simulink model "VDSE_2018b"  (R2018b)
settings: Solver=ode5  StartTime=0.0  StopTime=T_simulation  FixedStep=simulation_step_time  RelTol=1e-3
values from neighbouring files (symbols this model uses):
  A = 2    [vehicle_parameters_script.m]
  bump_height = 0    [vehicle_parameters_script.m]
  bump_length = 1    [vehicle_parameters_script.m]
  bump_time = 1    [vehicle_parameters_script.m]
  Bxf = 17.156    [BCD_Parameters.m]
  Bxr = 17.156    [BCD_Parameters.m]
  Byf = 12.71    [BCD_Parameters.m]
  Byr = 12.71    [BCD_Parameters.m]
  cd = 0.35    [vehicle_parameters_script.m]
  central_diff = 1    [vehicle_parameters_script.m]
  cF = 5000    [vehicle_parameters_script.m]
  clF = -0.15    [vehicle_parameters_script.m]
  clR = -0.20    (= -0.2)    [vehicle_parameters_script.m]
  cp_FA = 30    [vehicle_parameters_script.m]
  cp_RA = 13    [vehicle_parameters_script.m]
  cR = 5000    [vehicle_parameters_script.m]
  ctF = tireF.VERTICAL_DAMPING    [vehicle_parameters_script.m]
  ctR = tireR.VERTICAL_DAMPING    [vehicle_parameters_script.m]
  Cxf = 1.406    [BCD_Parameters.m]
  Cxr = 1.406    [BCD_Parameters.m]
  Cyf = 1.63    [BCD_Parameters.m]
  Cyr = 1.63    [BCD_Parameters.m]
  Dxf = 1.2    [BCD_Parameters.m]
  Dxr = 1.2    [BCD_Parameters.m]
  Dyf = 1.1    [BCD_Parameters.m]
  Dyr = 1.8    [BCD_Parameters.m]
  enableDriverControl = 0    [vehicle_parameters_script.m]
  enableLongDynamics = 1    [vehicle_parameters_script.m]
  enablePowertrain = 1    [vehicle_parameters_script.m]
  front_dr = 3.8    [vehicle_parameters_script.m]
  g = 9.806    [vehicle_parameters_script.m]
  Gear_numbers = [1 2 3 4 5 6]    [vehicle_parameters_script.m]
  GR = [2.9 1.8 1.3 1 0.85 0.75]    [vehicle_parameters_script.m]
  hcog = 0.5    [vehicle_parameters_script.m]
  hpc = 0.0    (= 0)    [vehicle_parameters_script.m]
  hrcF = 0.3    [vehicle_parameters_script.m]
  hrcg = (hrcF*lR+hrcR*lF)/(lF+lR)    (= 0.25108)    [vehicle_parameters_script.m]
  hrcR = 0.2    [vehicle_parameters_script.m]
  huFcog = 0.32    [vehicle_parameters_script.m]
  huRcog = 0.32    [vehicle_parameters_script.m]
  initial_gear = 1    [vehicle_parameters_script.m]
  JwF = 2.45    [vehicle_parameters_script.m]
  JwR = 2.45    [vehicle_parameters_script.m]
  Jx = 430    [vehicle_parameters_script.m]
  Jy = 1309    [vehicle_parameters_script.m]
  Jz = 1461    [vehicle_parameters_script.m]
  kF = 40000    [vehicle_parameters_script.m]
  kR = 35000    [vehicle_parameters_script.m]
  kRF = 0    [vehicle_parameters_script.m]
  kRR = 0    [vehicle_parameters_script.m]
  ktF = tireF.VERTICAL_STIFFNESS    [vehicle_parameters_script.m]
  ktR = tireR.VERTICAL_STIFFNESS    [vehicle_parameters_script.m]
  lF = 1.223    [vehicle_parameters_script.m]
  lR = l-lF    (= 1.277)    [vehicle_parameters_script.m]
  m = 1310    [vehicle_parameters_script.m]
  max_pressure = 1000    [vehicle_parameters_script.m]
  maxrpm = 4000    [vehicle_parameters_script.m]
  mF = 45    [vehicle_parameters_script.m]
  minrpm = 1500    [vehicle_parameters_script.m]
  mR = 50    [vehicle_parameters_script.m]
  output_samping_time = 0.001    [vehicle_parameters_script.m]
  phi0 = 0    [vehicle_parameters_script.m]
  phi_dot0 = 0    [vehicle_parameters_script.m]
  psi0 = 0    [vehicle_parameters_script.m]
  psi_dot0 = 0    [vehicle_parameters_script.m]
  rear_dr = 3.8    [vehicle_parameters_script.m]
  requested_speed = 100/3.6    (= 27.7777777778)    [vehicle_parameters_script.m]
  rF = tireF.UNLOADED_RADIUS    [vehicle_parameters_script.m]
  rho = 1.2    [vehicle_parameters_script.m]
  RPMME = Engine(:,1)    [vehicle_parameters_script.m]
  rR = tireR.UNLOADED_RADIUS    [vehicle_parameters_script.m]
  steer_ratio = 13.25    [vehicle_parameters_script.m]
  TFL = 0    [vehicle_parameters_script.m]
  TFR = 0    [vehicle_parameters_script.m]
  theta0 = 0    [vehicle_parameters_script.m]
  theta_dot0 = 0    [vehicle_parameters_script.m]
  TorqueME = []    [vehicle_parameters_script.m]
  TRL = 0    [vehicle_parameters_script.m]
  TRR = 0    [vehicle_parameters_script.m]
  Vx0 = 100/3.6    (= 27.7777777778)    [vehicle_parameters_script.m]
  Vy0 = 0    [vehicle_parameters_script.m]
  Vz0 = 0    [vehicle_parameters_script.m]
  wF = 1.578    [vehicle_parameters_script.m]
  wR = 1.544    [vehicle_parameters_script.m]
  x0 = 0    [vehicle_parameters_script.m]
  xcog_overall = (2*mR*xR+2*xF*mF+m*xs)/(m+2*mF+2*mR)    (= 1.23475333333)    [vehicle_parameters_script.m]
  y0 = 0    [vehicle_parameters_script.m]
  z0 = 0    [vehicle_parameters_script.m]
  zFL0 = 0    [vehicle_parameters_script.m]
  zFL_dot0 = 0    [vehicle_parameters_script.m]
  zFR0 = 0    [vehicle_parameters_script.m]
  zFR_dot0 = 0    [vehicle_parameters_script.m]
  zRL0 = 0    [vehicle_parameters_script.m]
  zRL_dot0 = 0    [vehicle_parameters_script.m]
  zRR0 = 0    [vehicle_parameters_script.m]
  zRR_dot0 = 0    [vehicle_parameters_script.m]
undefined symbols (not defined in the file or in its folder): exf, exr, eyf, eyr, FNOMINf, FNOMINr, PCX1f, PCX1r, PCY1f, PCY1r, PDX1f, PDX1r, PDX2f, PDX2r, PDY1f, PDY1r, PDY2f, PDY2r, PDY3f, PDY3r, PEX1f, PEX1r, PEX2f, PEX2r, PEX3f, PEX3r, PEX4f, PEX4r, PEY1f, PEY1r, PEY2f, PEY2r, PEY3f, PEY3r, PEY4f, PEY4r, PHX1f, PHX1r, PHX2f, PHX2r, PHY1f, PHY1r, PHY2f, PHY2r, PHY3f, PHY3r, PKX1f, PKX1r, PKX2f, PKX2r, PKX3f, PKX3r, PKY1f, PKY1r, PKY2f, PKY2r, PKY3f, PKY3r, PVX1f, PVX1r ... (+122)
libraries: simulink x7, mfeval_LIB x4
(part 2 of 6)

== system VDSE_2018b/14-DOF VEHICLE MODEL/EQUATIONS OF MOTION FOR CHASSIS/Lateral Dynamics ==
  deltaFL [rad] : Inport
  deltaFR [rad] : Inport  Port=2
  delta RL [rad] : Inport  Port=3
  delta RR [rad] : Inport  Port=4
  fFLx [N] : Inport  Port=5
  fFRx [N] : Inport  Port=6
  fRLx [N] : Inport  Port=7
  fRRx [N] : Inport  Port=8
  fFLy [N] : Inport  Port=9
  fFRy [N] : Inport  Port=10
  fRLy [N] : Inport  Port=11
  fRRy [N] : Inport  Port=12
  mFLy [Nm] : Inport  Port=13
  mFRy [Nm] : Inport  Port=14
  mRLy [Nm] : Inport  Port=15
  mRRy [Nm] : Inport  Port=16
  Vx [m/s] : Inport  Port=17
  psi_dot [rad/s] : Inport  Port=18
  phi_dot [rad/s] : Inport  Port=19
  Vz [m/s] : Inport  Port=20
  Constant : Constant  Value=y0
  Constant1 : Constant  Value=Vy0
  Constant2 : Constant  Value=m
  Constant3 : Constant  Value=mF
  Constant4 : Constant  Value=mR
  Constant5 : Constant  Value=rF
  Constant6 : Constant  Value=rR
  Integrator : Integrator  InitialConditionSource=external
  Integrator1 : Integrator  InitialConditionSource=external
  LATERAL DYNAMICS : MATLAB Function  TreatAsAtomicUnit=on
  ay [m/s^2] : Outport
  Vy [m/s] : Outport  Port=2
  lateral y [m] : Outport  Port=3
  wires:
  Integrator/1 -> lateral y [m]/1  "y"
  Constant/1 -> Integrator/2
  Integrator1/1 -> Vy [m/s]/1, Integrator/1  "Vy"
  Constant1/1 -> Integrator1/2
  LATERAL DYNAMICS/2(Vy_dot) -> Integrator1/1  "Vy_dot"
  Vx [m/s]/1 -> LATERAL DYNAMICS/17(Vx)
  LATERAL DYNAMICS/1(ay) -> ay [m/s^2]/1  "ay"
  deltaFL [rad]/1 -> LATERAL DYNAMICS/1(deltaFL)
  fFLx [N]/1 -> LATERAL DYNAMICS/2(fFLx)
  fFLy [N]/1 -> LATERAL DYNAMICS/3(fFLy)
  deltaFR [rad]/1 -> LATERAL DYNAMICS/4(deltaFR)
  fFRx [N]/1 -> LATERAL DYNAMICS/5(fFRx)
  fFRy [N]/1 -> LATERAL DYNAMICS/6(fFRy)
  delta RL [rad]/1 -> LATERAL DYNAMICS/7(deltaRL)
  fRLx [N]/1 -> LATERAL DYNAMICS/8(fRLx)
  fRLy [N]/1 -> LATERAL DYNAMICS/9(fRLy)
  delta RR [rad]/1 -> LATERAL DYNAMICS/10(deltaRR)
  fRRx [N]/1 -> LATERAL DYNAMICS/11(fRRx)
  fRRy [N]/1 -> LATERAL DYNAMICS/12(fRRy)
  psi_dot [rad/s]/1 -> LATERAL DYNAMICS/18(psi_dot)
  phi_dot [rad/s]/1 -> LATERAL DYNAMICS/19(phi_dot)
  Vz [m/s]/1 -> LATERAL DYNAMICS/20(Vz)
  Constant2/1 -> LATERAL DYNAMICS/21(m)
  Constant3/1 -> LATERAL DYNAMICS/22(mF)
  Constant4/1 -> LATERAL DYNAMICS/23(mR)
  Constant5/1 -> LATERAL DYNAMICS/24(rF)
  Constant6/1 -> LATERAL DYNAMICS/25(rR)
  mFLy [Nm]/1 -> LATERAL DYNAMICS/13(mFLy)
  mFRy [Nm]/1 -> LATERAL DYNAMICS/14(mFRy)
  mRLy [Nm]/1 -> LATERAL DYNAMICS/15(mRLy)
  mRRy [Nm]/1 -> LATERAL DYNAMICS/16(mRRy)

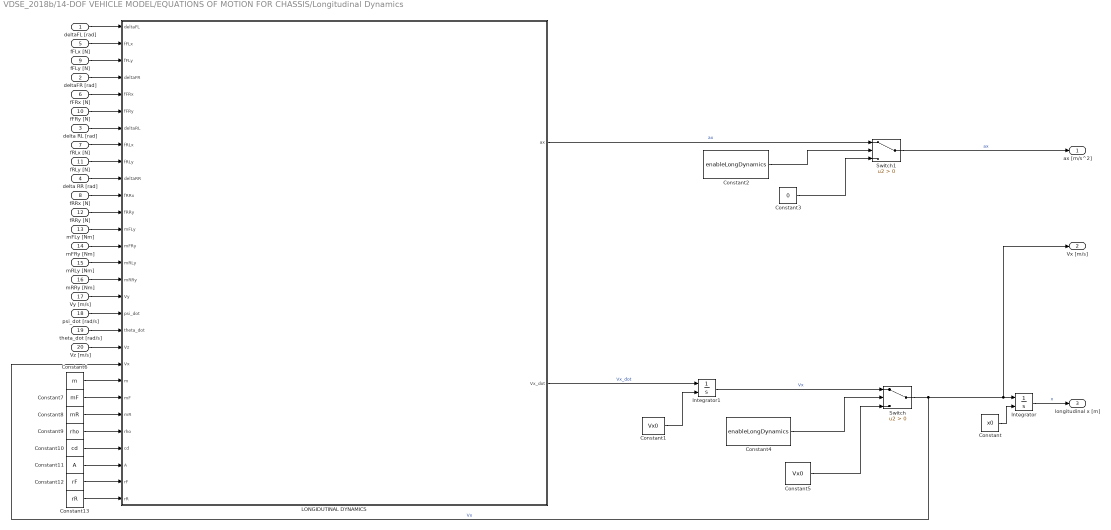
== system VDSE_2018b/14-DOF VEHICLE MODEL/EQUATIONS OF MOTION FOR CHASSIS/Longitudinal Dynamics ==
  deltaFL [rad] : Inport
  deltaFR [rad] : Inport  Port=2
  delta RL [rad] : Inport  Port=3
  delta RR [rad] : Inport  Port=4
  fFLx [N] : Inport  Port=5
  fFRx [N] : Inport  Port=6
  fRLx [N] : Inport  Port=7
  fRRx [N] : Inport  Port=8
  fFLy [N] : Inport  Port=9
  fFRy [N] : Inport  Port=10
  fRLy [N] : Inport  Port=11
  fRRy [N] : Inport  Port=12
  mFLy [Nm] : Inport  Port=13
  mFRy [Nm] : Inport  Port=14
  mRLy [Nm] : Inport  Port=15
  mRRy [Nm] : Inport  Port=16
  Vy [m/s] : Inport  Port=17
  psi_dot [rad/s] : Inport  Port=18
  theta_dot [rad/s] : Inport  Port=19
  Vz [m/s] : Inport  Port=20
  Constant : Constant  Value=x0
  Constant1 : Constant  Value=Vx0
  Constant10 : Constant  Value=cd
  Constant11 : Constant  Value=A
  Constant12 : Constant  Value=rF
  Constant13 : Constant  Value=rR
  Constant2 : Constant  Value=enableLongDynamics
  Constant3 : Constant  Value=0
  Constant4 : Constant  Value=enableLongDynamics
  Constant5 : Constant  Value=Vx0
  Constant6 : Constant  Value=m
  Constant7 : Constant  Value=mF
  Constant8 : Constant  Value=mR
  Constant9 : Constant  Value=rho
  Integrator : Integrator  InitialConditionSource=external
  Integrator1 : Integrator  InitialConditionSource=external
  LONGIDUTINAL DYNAMICS : MATLAB Function  TreatAsAtomicUnit=on
  Switch : Switch  Criteria=u2 > Threshold
  Switch1 : Switch  Criteria=u2 > Threshold
  ax [m/s^2] : Outport
  Vx [m/s] : Outport  Port=2
  longitudinal x [m] : Outport  Port=3
  wires:
  LONGIDUTINAL DYNAMICS/2(Vx_dot) -> Integrator1/1  "Vx_dot"
  Constant1/1 -> Integrator1/2
  Constant/1 -> Integrator/2
  Integrator/1 -> longitudinal x [m]/1  "x"
  Constant4/1 -> Switch/2
  Constant5/1 -> Switch/3
  Switch1/1 -> ax [m/s^2]/1  "ax"
  Constant3/1 -> Switch1/3
  Constant2/1 -> Switch1/2
  Switch/1 -> Vx [m/s]/1, Integrator/1, LONGIDUTINAL DYNAMICS/21(Vx)  "Vx"
  deltaFL [rad]/1 -> LONGIDUTINAL DYNAMICS/1(deltaFL)
  fFLx [N]/1 -> LONGIDUTINAL DYNAMICS/2(fFLx)
  fFLy [N]/1 -> LONGIDUTINAL DYNAMICS/3(fFLy)
  deltaFR [rad]/1 -> LONGIDUTINAL DYNAMICS/4(deltaFR)
  fFRx [N]/1 -> LONGIDUTINAL DYNAMICS/5(fFRx)
  fFRy [N]/1 -> LONGIDUTINAL DYNAMICS/6(fFRy)
  delta RL [rad]/1 -> LONGIDUTINAL DYNAMICS/7(deltaRL)
  fRLx [N]/1 -> LONGIDUTINAL DYNAMICS/8(fRLx)
  fRLy [N]/1 -> LONGIDUTINAL DYNAMICS/9(fRLy)
  delta RR [rad]/1 -> LONGIDUTINAL DYNAMICS/10(deltaRR)
  fRRx [N]/1 -> LONGIDUTINAL DYNAMICS/11(fRRx)
  fRRy [N]/1 -> LONGIDUTINAL DYNAMICS/12(fRRy)
  Vy [m/s]/1 -> LONGIDUTINAL DYNAMICS/17(Vy)
  psi_dot [rad/s]/1 -> LONGIDUTINAL DYNAMICS/18(psi_dot)
  theta_dot [rad/s]/1 -> LONGIDUTINAL DYNAMICS/19(theta_dot)
  Vz [m/s]/1 -> LONGIDUTINAL DYNAMICS/20(Vz)
  Constant6/1 -> LONGIDUTINAL DYNAMICS/22(m)
  Constant7/1 -> LONGIDUTINAL DYNAMICS/23(mF)
  Constant8/1 -> LONGIDUTINAL DYNAMICS/24(mR)
  Constant9/1 -> LONGIDUTINAL DYNAMICS/25(rho)
  Constant10/1 -> LONGIDUTINAL DYNAMICS/26(cd)
  Constant11/1 -> LONGIDUTINAL DYNAMICS/27(A)
  Integrator1/1 -> Switch/1  "Vx"
  LONGIDUTINAL DYNAMICS/1(ax) -> Switch1/1  "ax"
  mFLy [Nm]/1 -> LONGIDUTINAL DYNAMICS/13(mFLy)
  mFRy [Nm]/1 -> LONGIDUTINAL DYNAMICS/14(mFRy)
  mRLy [Nm]/1 -> LONGIDUTINAL DYNAMICS/15(mRLy)
  mRRy [Nm]/1 -> LONGIDUTINAL DYNAMICS/16(mRRy)
  Constant12/1 -> LONGIDUTINAL DYNAMICS/28(rF)
  Constant13/1 -> LONGIDUTINAL DYNAMICS/29(rR)

== system VDSE_2018b/14-DOF VEHICLE MODEL/EQUATIONS OF MOTION FOR CHASSIS/Pitch Dynamics ==
  Vz [m/s] : Inport
  zFL_dot [m/s] : Inport  Port=2
  zFR_dot [m/s] : Inport  Port=3
  zRR_dot [m/s] : Inport  Port=4
  zRL_dot [m/s] : Inport  Port=5
  phi_dot [rad/s] : Inport  Port=6
  z [m] : Inport  Port=7
  zFL [m] : Inport  Port=8
  zFR [m] : Inport  Port=9
  zRR [m] : Inport  Port=10
  zRL [m] : Inport  Port=11
  phi [rad] : Inport  Port=12
  ax [m/s^2] : Inport  Port=13
  Vx [m/s] : Inport  Port=14
  Constant : Constant  Value=theta0
  Constant1 : Constant  Value=theta_dot0
  Constant10 : Constant  Value=kR
  Constant11 : Constant  Value=cF
  Constant12 : Constant  Value=cR
  Constant13 : Constant  Value=m
  Constant14 : Constant  Value=hcog
  Constant2 : Constant  Value=Jy
  Constant3 : Constant  Value=g
  Constant4 : Constant  Value=hpc
  Constant5 : Constant  Value=lF
  Constant6 : Constant  Value=lR
  Constant7 : Constant  Value=wF
  Constant8 : Constant  Value=wR
  Constant9 : Constant  Value=kF
  Downforce : Subsystem
  Integrator : Integrator  InitialConditionSource=external
  Integrator1 : Integrator  InitialConditionSource=external
  PITCH DYNAMICS : MATLAB Function  TreatAsAtomicUnit=on
  theta_dot_dot [rad/s^2] : Outport
  theta_dot [rad/s] : Outport  Port=2
  theta [rad] : Outport  Port=3
  wires:
  Constant1/1 -> Integrator1/2
  Integrator1/1 -> theta_dot [rad/s]/1, Integrator/1, PITCH DYNAMICS/32(theta_dot)  "theta_dot"
  Constant/1 -> Integrator/2
  Integrator/1 -> theta [rad]/1, PITCH DYNAMICS/31(theta)  "theta"
  ax [m/s^2]/1 -> PITCH DYNAMICS/23(ax)
  Constant6/1 -> PITCH DYNAMICS/4(lR)
  Constant7/1 -> PITCH DYNAMICS/5(wF)
  Constant10/1 -> PITCH DYNAMICS/8(kR)
  Constant9/1 -> PITCH DYNAMICS/7(kF)
  Constant2/1 -> PITCH DYNAMICS/1(Jy)
  Constant5/1 -> PITCH DYNAMICS/3(lF)
  Constant11/1 -> PITCH DYNAMICS/9(cF)
  Constant8/1 -> PITCH DYNAMICS/6(wR)
  Constant3/1 -> PITCH DYNAMICS/2(g)
  PITCH DYNAMICS/1(theta_dot_dot) -> theta_dot_dot [rad/s^2]/1, Integrator1/1  "theta_dot_dot"
  Vz [m/s]/1 -> PITCH DYNAMICS/12(z_dot)
  Constant12/1 -> PITCH DYNAMICS/10(cR)
  zFL_dot [m/s]/1 -> PITCH DYNAMICS/16(zFL_dot)
  zFR_dot [m/s]/1 -> PITCH DYNAMICS/18(zFR_dot)
  zRR_dot [m/s]/1 -> PITCH DYNAMICS/22(zRR_dot)
  zRL_dot [m/s]/1 -> PITCH DYNAMICS/20(zRL_dot)
  phi_dot [rad/s]/1 -> PITCH DYNAMICS/14(phi_dot)
  z [m]/1 -> PITCH DYNAMICS/11(z)
  phi [rad]/1 -> PITCH DYNAMICS/13(phi)
  zFL [m]/1 -> PITCH DYNAMICS/15(zFL)
  zFR [m]/1 -> PITCH DYNAMICS/17(zFR)
  zRR [m]/1 -> PITCH DYNAMICS/21(zRR)
  zRL [m]/1 -> PITCH DYNAMICS/19(zRL)
  Constant4/1 -> PITCH DYNAMICS/24(hpc)
  Constant13/1 -> PITCH DYNAMICS/26(m)
  Constant14/1 -> PITCH DYNAMICS/25(hcog)
  Downforce/1(fFLz_overall) -> PITCH DYNAMICS/27(fFLz_aero)  "FLz_overall_aero"
  Downforce/2(fFRz_overall) -> PITCH DYNAMICS/28(fFRz_aero)  "FRz_overall_aero"
  Downforce/3(fRLz_overall) -> PITCH DYNAMICS/29(fRLz_aero)  "RLz_overall_aero"
  Vx [m/s]/1 -> Downforce/1(Vx)
  Downforce/4(fRRz_overall) -> PITCH DYNAMICS/30(fRRz_aero)  "RRz_overall_aero"

== system VDSE_2018b/14-DOF VEHICLE MODEL/EQUATIONS OF MOTION FOR CHASSIS/Roll Dynamics ==
  Vz[m/s] : Inport
  zFL_dot [m/s^2] : Inport  Port=2
  zFR_dot [m/s^2] : Inport  Port=3
  zRR_dot [m/s^2] : Inport  Port=4
  zRL_dot [m/s^2] : Inport  Port=5
  theta_dot [rad/s] : Inport  Port=6
  z [m] : Inport  Port=7
  zFL [m] : Inport  Port=8
  zFR [m] : Inport  Port=9
  zRR [m] : Inport  Port=10
  zRL [m] : Inport  Port=11
  theta [rad] : Inport  Port=12
  ay [m/s^2] : Inport  Port=13
  Vx [m/s] : Inport  Port=14
  Constant : Constant  Value=phi0
  Constant1 : Constant  Value=phi_dot0
  Constant10 : Constant  Value=kR
  Constant11 : Constant  Value=cF
  Constant12 : Constant  Value=cR
  Constant13 : Constant  Value=kRF
  Constant14 : Constant  Value=hrcg
  Constant15 : Constant  Value=m
  Constant16 : Constant  Value=hcog
  Constant2 : Constant  Value=Jx
  Constant3 : Constant  Value=g
  Constant4 : Constant  Value=kRR
  Constant5 : Constant  Value=lF
  Constant6 : Constant  Value=lR
  Constant7 : Constant  Value=wF
  Constant8 : Constant  Value=wR
  Constant9 : Constant  Value=kF
  Downforce : Subsystem
  Integrator : Integrator  InitialConditionSource=external
  Integrator1 : Integrator  InitialConditionSource=external
  ROLL DYNAMICS : MATLAB Function  TreatAsAtomicUnit=on
  phi_dot_dot [rad/s^2] : Outport
  phi_dot [rad/s] : Outport  Port=2
  phi [rad] : Outport  Port=3
  wires:
  Constant/1 -> Integrator/2
  Integrator1/1 -> phi_dot [rad/s]/1, Integrator/1, ROLL DYNAMICS/34(phi_dot)  "phi_dot"
  Constant1/1 -> Integrator1/2
  Integrator/1 -> phi [rad]/1, ROLL DYNAMICS/33(phi)  "phi"
  Constant11/1 -> ROLL DYNAMICS/11(cF)
  Constant10/1 -> ROLL DYNAMICS/8(kR)
  Constant2/1 -> ROLL DYNAMICS/1(Jx)
  Constant12/1 -> ROLL DYNAMICS/12(cR)
  Constant3/1 -> ROLL DYNAMICS/2(g)
  Constant5/1 -> ROLL DYNAMICS/3(lF)
  Constant6/1 -> ROLL DYNAMICS/4(lR)
  Constant13/1 -> ROLL DYNAMICS/9(kRF)
  Constant4/1 -> ROLL DYNAMICS/10(kRR)
  Constant7/1 -> ROLL DYNAMICS/5(wF)
  Constant8/1 -> ROLL DYNAMICS/6(wR)
  Constant9/1 -> ROLL DYNAMICS/7(kF)
  ROLL DYNAMICS/1(phi_dot_dot) -> Integrator1/1, phi_dot_dot [rad/s^2]/1  "phi_dot_dot"
  z [m]/1 -> ROLL DYNAMICS/13(z)
  Vz[m/s]/1 -> ROLL DYNAMICS/14(z_dot)
  theta_dot [rad/s]/1 -> ROLL DYNAMICS/16(theta_dot)
  theta [rad]/1 -> ROLL DYNAMICS/15(theta)
  zFL [m]/1 -> ROLL DYNAMICS/17(zFL)
  zFR [m]/1 -> ROLL DYNAMICS/19(zFR)
  zRR [m]/1 -> ROLL DYNAMICS/23(zRR)
  zRL [m]/1 -> ROLL DYNAMICS/21(zRL)
  zRL_dot [m/s^2]/1 -> ROLL DYNAMICS/22(zRL_dot)
  zRR_dot [m/s^2]/1 -> ROLL DYNAMICS/24(zRR_dot)
  zFR_dot [m/s^2]/1 -> ROLL DYNAMICS/20(zFR_dot)
  zFL_dot [m/s^2]/1 -> ROLL DYNAMICS/18(zFL_dot)
  ay [m/s^2]/1 -> ROLL DYNAMICS/25(ay)
  Constant14/1 -> ROLL DYNAMICS/26(hrcg)
  Constant15/1 -> ROLL DYNAMICS/28(m)
  Constant16/1 -> ROLL DYNAMICS/27(hcog)
  Vx [m/s]/1 -> Downforce/1(Vx)
  Downforce/1(fFLz_overall) -> ROLL DYNAMICS/29(fFLz_aero)  "FLz_overall_aero"
  Downforce/2(fFRz_overall) -> ROLL DYNAMICS/30(fFRz_aero)  "FRz_overall_aero"
  Downforce/3(fRLz_overall) -> ROLL DYNAMICS/31(fRLz_aero)  "RLz_overall_aero"
  Downforce/4(fRRz_overall) -> ROLL DYNAMICS/32(fRRz_aero)  "RRz_overall_aero"

== system VDSE_2018b/14-DOF VEHICLE MODEL/EQUATIONS OF MOTION FOR CHASSIS/Vertical Dynamics ==
  zFL_dot [m/s] : Inport
  ZFR_dot [m/s] : Inport  Port=2
  zRR_dot [m/s] : Inport  Port=3
  zRL_dot [m/s] : Inport  Port=4
  Vx [m/s] : Inport  Port=5
  theta_dot [rad/s] : Inport  Port=6
  phi_dot [rad/s] : Inport  Port=7
  Vy [m/s] : Inport  Port=8
  zFL [m] : Inport  Port=9
  zFR [m] : Inport  Port=10
  zRR [m] : Inport  Port=11
  zRL [m] : Inport  Port=12
  theta [rad] : Inport  Port=13
  phi [rad] : Inport  Port=14
  Constant : Constant  Value=z0
  Constant1 : Constant  Value=Vz0
  Constant10 : Constant  Value=kR
  Constant11 : Constant  Value=cF
  Constant12 : Constant  Value=cR
  Constant2 : Constant  Value=m
  Constant3 : Constant  Value=g
  Constant5 : Constant  Value=lF
  Constant6 : Constant  Value=lR
  Constant7 : Constant  Value=wF
  Constant8 : Constant  Value=wR
  Constant9 : Constant  Value=kF
  Downforce : Subsystem
  Integrator : Integrator  InitialConditionSource=external
  Integrator1 : Integrator  InitialConditionSource=external
  VERTICAL DYNAMICS : MATLAB Function  TreatAsAtomicUnit=on
  Vx [m/s]1 : InportShadow  Port=5
  Vz_dot [m/s^2] : Outport
  Vz [m/s] : Outport  Port=2
  vertical z [m] : Outport  Port=3
  wires:
  phi_dot [rad/s]/1 -> VERTICAL DYNAMICS/12(phi_dot)
  theta_dot [rad/s]/1 -> VERTICAL DYNAMICS/14(theta_dot)
  VERTICAL DYNAMICS/1(Vz_dot) -> Integrator1/1, Vz_dot [m/s^2]/1  "Vz_dot"
  Constant1/1 -> Integrator1/2
  Integrator1/1 -> Vz [m/s]/1, Integrator/1, VERTICAL DYNAMICS/30(z_dot)  "Vz"
  Constant/1 -> Integrator/2
  Constant12/1 -> VERTICAL DYNAMICS/10(cR)
  Constant11/1 -> VERTICAL DYNAMICS/9(cF)
  Constant10/1 -> VERTICAL DYNAMICS/8(kR)
  Constant9/1 -> VERTICAL DYNAMICS/7(kF)
  Constant8/1 -> VERTICAL DYNAMICS/6(wR)
  Constant7/1 -> VERTICAL DYNAMICS/5(wF)
  Constant6/1 -> VERTICAL DYNAMICS/4(lR)
  Constant5/1 -> VERTICAL DYNAMICS/3(lF)
  Constant3/1 -> VERTICAL DYNAMICS/2(g)
  Constant2/1 -> VERTICAL DYNAMICS/1(m)
  phi [rad]/1 -> VERTICAL DYNAMICS/11(phi)
  theta [rad]/1 -> VERTICAL DYNAMICS/13(theta)
  zFL_dot [m/s]/1 -> VERTICAL DYNAMICS/16(zFL_dot)
  ZFR_dot [m/s]/1 -> VERTICAL DYNAMICS/18(zFR_dot)
  zRR_dot [m/s]/1 -> VERTICAL DYNAMICS/22(zRR_dot)
  zRL_dot [m/s]/1 -> VERTICAL DYNAMICS/20(zRL_dot)
  zFL [m]/1 -> VERTICAL DYNAMICS/15(zFL)
  zFR [m]/1 -> VERTICAL DYNAMICS/17(zFR)
  zRR [m]/1 -> VERTICAL DYNAMICS/21(zRR)
  zRL [m]/1 -> VERTICAL DYNAMICS/19(zRL)
  Integrator/1 -> vertical z [m]/1, VERTICAL DYNAMICS/29(z)  "z"
  Vy [m/s]/1 -> VERTICAL DYNAMICS/24(Vy)
  Vx [m/s]/1 -> VERTICAL DYNAMICS/23(Vx)
  Downforce/1(fFLz_overall) -> VERTICAL DYNAMICS/25(fFLz_aero)  "FLz_overall_aero"
  Downforce/2(fFRz_overall) -> VERTICAL DYNAMICS/26(fFRz_aero)  "FRz_overall_aero"
  Downforce/3(fRLz_overall) -> VERTICAL DYNAMICS/27(fRLz_aero)  "RLz_overall_aero"
  Downforce/4(fRRz_overall) -> VERTICAL DYNAMICS/28(fRRz_aero)  "RRz_overall_aero"
  Vx [m/s]1/1 -> Downforce/1(Vx)

== system VDSE_2018b/14-DOF VEHICLE MODEL/EQUATIONS OF MOTION FOR CHASSIS/Yaw Dynamics ==
  fFLy [N] : Inport
  fFRy [N] : Inport  Port=2
  fRLy [N] : Inport  Port=3
  fRRy [N] : Inport  Port=4
  fFLx [N] : Inport  Port=5
  fFRx [N] : Inport  Port=6
  fRLx [N] : Inport  Port=7
  fRRx [N] : Inport  Port=8
  deltaFL [rad] : Inport  Port=9
  deltaFR [rad] : Inport  Port=10
  deltaRL [rad] : Inport  Port=11
  deltaRR [rad] : Inport  Port=12
  mFLz : Inport  Port=13
  mFRz : Inport  Port=14
  mRLz : Inport  Port=15
  mRRz : Inport  Port=16
  Constant : Constant  Value=psi0
  Constant1 : Constant  Value=psi_dot0
  Constant2 : Constant  Value=mF
  Constant3 : Constant  Value=mR
  Constant4 : Constant  Value=xcog_overall
  Constant5 : Constant  Value=l-xcog_overall
  Constant6 : Constant  Value=wF
  Constant7 : Constant  Value=wR
  Constant8 : Constant  Value=Jz
  Integrator : Integrator  InitialConditionSource=external
  Integrator1 : Integrator  InitialConditionSource=external
  YAW DYNAMICS : MATLAB Function  TreatAsAtomicUnit=on
  psi_dot_dot [rad/s^2] : Outport
  psi_dot [rad/s] : Outport  Port=2
  psi [rad] : Outport  Port=3
  wires:
  Integrator/1 -> psi [rad]/1  "psi"
  Constant/1 -> Integrator/2
  Integrator1/1 -> psi_dot [rad/s]/1, Integrator/1  "psi_dot"
  Constant1/1 -> Integrator1/2
  YAW DYNAMICS/1(psi_dot_dot) -> psi_dot_dot [rad/s^2]/1, Integrator1/1  "psi_dot_dot"
  mFLz/1 -> YAW DYNAMICS/14(mFLz)
  mFRz/1 -> YAW DYNAMICS/15(mFRz)
  mRLz/1 -> YAW DYNAMICS/16(mRLz)
  mRRz/1 -> YAW DYNAMICS/17(mRRz)
  Constant6/1 -> YAW DYNAMICS/18(wF)
  Constant7/1 -> YAW DYNAMICS/19(wR)
  Constant2/1 -> YAW DYNAMICS/20(mF)
  Constant3/1 -> YAW DYNAMICS/21(mR)
  Constant4/1 -> YAW DYNAMICS/22(lF)
  Constant5/1 -> YAW DYNAMICS/23(lR)
  Constant8/1 -> YAW DYNAMICS/24(Jz)
  [ay] -> YAW DYNAMICS/13(ay)
  fFLy [N]/1 -> YAW DYNAMICS/3(fFLy)
  fFRy [N]/1 -> YAW DYNAMICS/6(fFRy)
  deltaFL [rad]/1 -> YAW DYNAMICS/1(deltaFL)
  deltaFR [rad]/1 -> YAW DYNAMICS/4(deltaFR)
  fFLx [N]/1 -> YAW DYNAMICS/2(fFLx)
  fFRx [N]/1 -> YAW DYNAMICS/5(fFRx)
  deltaRL [rad]/1 -> YAW DYNAMICS/7(deltaRL)
  fRLx [N]/1 -> YAW DYNAMICS/8(fRLx)
  fRLy [N]/1 -> YAW DYNAMICS/9(fRLy)
  deltaRR [rad]/1 -> YAW DYNAMICS/10(deltaRR)
  fRRx [N]/1 -> YAW DYNAMICS/11(fRRx)
  fRRy [N]/1 -> YAW DYNAMICS/12(fRRy)

== system VDSE_2018b/14-DOF VEHICLE MODEL/POWERTRAIN AND BRAKES/Braking ==
  BRAKING [%] : Inport
  Bus Selector2 : BusSelector  OutputSignals=Throttle and Braking.Braking [%]
  Constant : Constant  Value=max_pressure
  Gain : Gain  Gain=-0.01
  Gain1 : Gain  Gain=cp_FA
  Gain2 : Gain  Gain=cp_RA
  Gain3 : Gain  Gain=0.5
  Gain4 : Gain  Gain=0.5
  Product{,1..4} (5 alike) : Product
  Saturation{,1..3} (4 alike) : Saturate  UpperLimit=1  LowerLimit=-1
  TBRAKE_FL_atWheels [Nm] : Outport
  TBRAKE_FR_atWheels [Nm] : Outport  Port=2
  TBRAKE_RL_atWheels [Nm] : Outport  Port=3
  TBRAKE_RR_atWheels [Nm] : Outport  Port=4
  tag scope: Braking=global, TBRAKE_FL_atWheels=global, TBRAKE_FR_atWheels=global, TBRAKE_RL_atWheels=global, TBRAKE_RR_atWheels=global
  wires:
  BRAKING [%]/1 -> Bus Selector2/1
  Bus Selector2/1 -> [Braking], Gain/1  "<Braking [%]>"
  Gain/1 -> Product/2
  Constant/1 -> Product/1
  Product/1 -> Gain2/1, Gain1/1
  Gain1/1 -> Gain3/1  "Tbrake_front [Nm]"
  Gain2/1 -> Gain4/1  "Tbrake_rear [Nm]"
  Gain3/1 -> Product2/2, Product1/2  "Tbrake_front_atWheels"
  Gain4/1 -> Product4/2, Product3/2  "Tbrake_rear_atWheels"
  Product1/1 -> TBRAKE_FL_atWheels [Nm]/1, [TBRAKE_FL_atWheels]  "FL"
  Product2/1 -> [TBRAKE_FR_atWheels], TBRAKE_FR_atWheels [Nm]/1
  Product3/1 -> TBRAKE_RL_atWheels [Nm]/1, [TBRAKE_RL_atWheels]
  Product4/1 -> [TBRAKE_RR_atWheels], TBRAKE_RR_atWheels [Nm]/1
  [omegaFL] -> Saturation/1
  [omegaFR] -> Saturation1/1
  [omegaRL] -> Saturation2/1
  [omegaRR] -> Saturation3/1
  Saturation/1 -> Product1/1
  Saturation1/1 -> Product2/1
  Saturation2/1 -> Product3/1
  Saturation3/1 -> Product4/1

== system VDSE_2018b/14-DOF VEHICLE MODEL/POWERTRAIN AND BRAKES/Enable Powertrain ==
  <TFL [Nm]> : Inport
  <TFR [Nm]> : Inport  Port=2
  <TRL [Nm]> : Inport  Port=3
  <TRR [Nm]> : Inport  Port=4
  Constant10 : Constant  Value=TFL
  Constant11 : Constant  Value=TFR
  Constant12 : Constant  Value=TRL
  Constant15 : Constant  Value=TRR
  Constant{16..19} (4 alike) : Constant  Value=enablePowertrain
  Switch{,1..3} (4 alike) : Switch  Criteria=u2 > Threshold
  TFL [Nm] : Outport
  TFR [Nm] : Outport  Port=2
  TRL [Nm] : Outport  Port=3
  TRR [Nm] : Outport  Port=4
  wires:
  Constant18/1 -> Switch/2
  Constant15/1 -> Switch3/3
  <TRR [Nm]>/1 -> Switch3/1
  Constant19/1 -> Switch3/2
  Switch/1 -> TFL [Nm]/1
  Constant10/1 -> Switch/3
  Constant17/1 -> Switch1/2
  <TFL [Nm]>/1 -> Switch/1
  Constant12/1 -> Switch2/3
  Constant11/1 -> Switch1/3
  Constant16/1 -> Switch2/2
  Switch2/1 -> TRL [Nm]/1
  Switch3/1 -> TRR [Nm]/1
  <TFR [Nm]>/1 -> Switch1/1
  <TRL [Nm]>/1 -> Switch2/1
  Switch1/1 -> TFR [Nm]/1

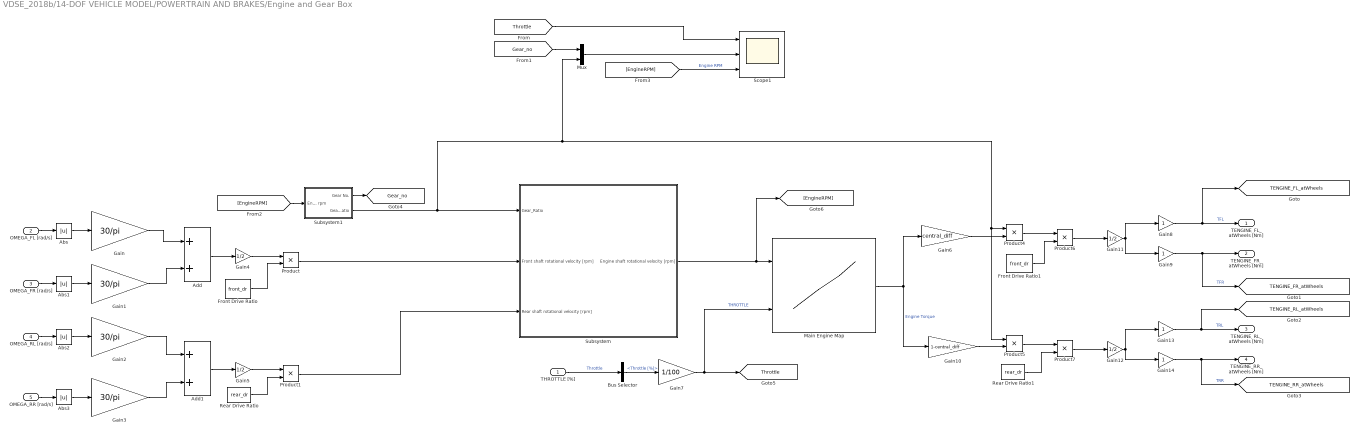
== system VDSE_2018b/14-DOF VEHICLE MODEL/POWERTRAIN AND BRAKES/Engine and Gear Box ==
  THROTTLE [%] : Inport
  OMEGA_FL [rad/s] : Inport  Port=2
  OMEGA_FR [rad/s] : Inport  Port=3
  OMEGA_RL [rad/s] : Inport  Port=4
  OMEGA_RR [rad/s] : Inport  Port=5
  Abs{,1..3} (4 alike) : Abs
  Add : Sum
  Add1 : Sum
  Bus Selector : BusSelector  OutputSignals=Throttle and Braking.Throttle [%]
  Front Drive Ratio : Constant  Value=front_dr
  Front Drive Ratio1 : Constant  Value=front_dr
  Gain{,1..3} (4 alike) : Gain  Gain=30/pi
  Gain10 : Gain  Gain=1-central_diff
  Gain{4..5,11..12} (4 alike) : Gain  Gain=1/2
  Gain{8..9,13..14} (4 alike) : Gain
  Gain6 : Gain  Gain=central_diff
  Gain7 : Gain  Gain=1/100
  Main Engine Map : Lookup_n-D  BreakpointsForDimension1=RPMME  BreakpointsForDimension2=[0:1/21:1]  Table=TorqueME  InterpMethod=Cubic spline  ExtrapMethod=Clip  InternalRulePriority=Speed  RndMeth=Simplest  InputSameDT=on
  Mux : Mux  Inputs=2
  Product{,1,4..7} (6 alike) : Product
  Rear Drive Ratio : Constant  Value=rear_dr
  Rear Drive Ratio1 : Constant  Value=rear_dr
  Scope1 : Scope  NumInputPorts=3
  Subsystem : Subsystem
  Subsystem1 : Subsystem
  TENGINE_FL_atWheels [Nm] : Outport
  TENGINE_FR_atWheels [Nm] : Outport  Port=2
  TENGINE_RL_atWheels [Nm] : Outport  Port=3
  TENGINE_RR_atWheels [Nm] : Outport  Port=4
  tag scope: Gear_no=global, TENGINE_FL_atWheels=global, TENGINE_FR_atWheels=global, TENGINE_RL_atWheels=global, TENGINE_RR_atWheels=global, Throttle=global
  wires:
  OMEGA_RL [rad/s]/1 -> Abs2/1
  OMEGA_RR [rad/s]/1 -> Abs3/1
  OMEGA_FR [rad/s]/1 -> Abs1/1
  OMEGA_FL [rad/s]/1 -> Abs/1
  Gain/1 -> Add/1
  Gain1/1 -> Add/2
  Add/1 -> Gain4/1
  Gain2/1 -> Add1/1
  Gain3/1 -> Add1/2
  Add1/1 -> Gain5/1
  Gain4/1 -> Product/1
  Front Drive Ratio/1 -> Product/2
  Gain5/1 -> Product1/1
  Rear Drive Ratio/1 -> Product1/2
  Bus Selector/1 -> Gain7/1  "<Throttle [%]>"
  Main Engine Map/1 -> Gain6/1, Gain10/1  "Engine Torque"
  Gain7/1 -> [Throttle], Main Engine Map/2  "THROTTLE"
  Abs/1 -> Gain/1
  Abs1/1 -> Gain1/1
  Abs2/1 -> Gain2/1
  Abs3/1 -> Gain3/1
  Gain10/1 -> Product5/2
  Gain6/1 -> Product4/2
  Rear Drive Ratio1/1 -> Product7/2
  Product5/1 -> Product7/1
  Front Drive Ratio1/1 -> Product6/2
  Product4/1 -> Product6/1
  Product6/1 -> Gain11/1
  Gain11/1 -> Gain8/1, Gain9/1
  Product7/1 -> Gain12/1
  Gain12/1 -> Gain13/1, Gain14/1
  Gain8/1 -> [TENGINE_FL_atWheels], TENGINE_FL_atWheels [Nm]/1  "TFL"
  Gain9/1 -> [TENGINE_FR_atWheels], TENGINE_FR_atWheels [Nm]/1  "TFR"
  Gain13/1 -> [TENGINE_RL_atWheels], TENGINE_RL_atWheels [Nm]/1  "TRL"
  Gain14/1 -> [TENGINE_RR_atWheels], TENGINE_RR_atWheels [Nm]/1  "TRR"
  THROTTLE [%]/1 -> Bus Selector/1  "Throttle"
  Product/1 -> Subsystem/2(Front shaft rotational velocity [rpm])
  Product1/1 -> Subsystem/3(Rear shaft rotational velocity [rpm])
  Subsystem/1(Engine shaft rotational velocity [rpm]) -> [EngineRPM], Main Engine Map/1
  Subsystem1/2(Gear_Ratio) -> Mux/2, Product5/1, Product4/1, Subsystem/1(Gear_Ratio)
  Mux/1 -> Scope1/2
  [Throttle] -> Scope1/1
  Subsystem1/1(Gear No.) -> [Gear_no]
  [Gear_no] -> Mux/1
  [EngineRPM] -> Subsystem1/1(Engine rpm)
  [EngineRPM] -> Scope1/3  "Engine RPM"

== system VDSE_2018b/14-DOF VEHICLE MODEL/POWERTRAIN AND BRAKES/Overall Torque Calculation ==
  TBRAKE_FL_atWheels [Nm] : Inport
  TBRAKE_FR_atWheels [Nm] : Inport  Port=2
  TBRAKE_RL_atWheels [Nm] : Inport  Port=3
  TBRAKE_RR_atWheels [Nm] : Inport  Port=4
  TENGINE_FL_atWheels [Nm] : Inport  Port=5
  TENGINE_FR_atWheels [Nm] : Inport  Port=6
  TENGINE_RL_atWheels [Nm] : Inport  Port=7
  TENGINE_RR_atWheels [Nm] : Inport  Port=8
  Add{,1..3} (4 alike) : Sum
  TFL [Nm] : Outport
  TFR [Nm] : Outport  Port=2
  TRL [Nm] : Outport  Port=3
  TRR [Nm] : Outport  Port=4
  wires:
  TENGINE_FL_atWheels [Nm]/1 -> Add/1
  TBRAKE_FL_atWheels [Nm]/1 -> Add/2
  TENGINE_FR_atWheels [Nm]/1 -> Add1/1
  Add3/1 -> TRR [Nm]/1  "TRR [Nm]"
  TBRAKE_RL_atWheels [Nm]/1 -> Add2/2
  TENGINE_RL_atWheels [Nm]/1 -> Add2/1
  Add2/1 -> TRL [Nm]/1  "TRL [Nm]"
  TENGINE_RR_atWheels [Nm]/1 -> Add3/1
  Add1/1 -> TFR [Nm]/1  "TFR [Nm]"
  Add/1 -> TFL [Nm]/1  "TFL [Nm]"
  TBRAKE_FR_atWheels [Nm]/1 -> Add1/2
  TBRAKE_RR_atWheels [Nm]/1 -> Add3/2

== system VDSE_2018b/14-DOF VEHICLE MODEL/SUSPENSION/FRONT SUSPENSION ==
  z [m] : Inport
  Vz [m/s] : Inport  Port=2
  phi [rad] : Inport  Port=3
  phi_dot [rad/s] : Inport  Port=4
  theta [rad] : Inport  Port=5
  theta_dot [rad/s] : Inport  Port=6
  yfront_road [m] : Inport  Port=7
  Bus Selector : BusSelector  OutputSignals=yFR_road [m]
  Bus Selector1 : BusSelector  OutputSignals=yFL_road [m]
  SUSPENSION FL : Subsystem
  SUSPENSION FR : Subsystem
  Vz [m/s]1 : InportShadow  Port=2
  phi [rad]1 : InportShadow  Port=3
  phi_dot [rad/s]1 : InportShadow  Port=4
  theta [rad]1 : InportShadow  Port=5
  theta_dot [rad/s]1 : InportShadow  Port=6
  yfront_road [m]1 : InportShadow  Port=7
  z [m]1 : InportShadow
  fFRz [N] : Outport
  fFLz [N] : Outport  Port=2
  zFR [m] : Outport  Port=3
  zFR_dot [m/s] : Outport  Port=4
  zFL [m] : Outport  Port=5
  zFL_dot [m/s] : Outport  Port=6
  wires:
  yfront_road [m]1/1 -> Bus Selector1/1  "yfront_road [m]"
  yfront_road [m]/1 -> Bus Selector/1  "yfront_road [m]"
  SUSPENSION FL/3(zFL [m]) -> [zFL], zFL [m]/1  "zFL [m]"
  SUSPENSION FL/2(zFL_dot [m/s]) -> zFL_dot [m/s]/1  "zFL_dot [m/s]"
  SUSPENSION FR/3(zFR_dot [m/s]) -> zFR_dot [m/s]/1  "zFR_dot [m/s]"
  SUSPENSION FR/2(zFR [m]) -> [zFR], zFR [m]/1  "zFR [m]"
  SUSPENSION FR/1(fFRz [N]) -> fFRz [N]/1  "fFRz [N]"
  SUSPENSION FL/1(fFLz [N]) -> fFLz [N]/1  "fFLz [N]"
  z [m]/1 -> SUSPENSION FR/1(z [m])  "z [m]"
  Vz [m/s]/1 -> SUSPENSION FR/2(Vz [m/s])  "Vz [m/s]"
  phi_dot [rad/s]/1 -> SUSPENSION FR/4(phi_dot [rad/s])  "phi_dot [rad/s]"
  phi [rad]/1 -> SUSPENSION FR/3(phi [rad])  "phi [rad]"
  theta [rad]/1 -> SUSPENSION FR/5(theta [rad])  "theta [rad]"
  theta_dot [rad/s]/1 -> SUSPENSION FR/6(theta_dot [rad/s])  "theta_dot [rad/s]"
  [zFL] -> SUSPENSION FR/7(zFL [m])
  [zFR] -> SUSPENSION FL/7(zFR [m])
  z [m]1/1 -> SUSPENSION FL/1(z [m])  "z [m]"
  Vz [m/s]1/1 -> SUSPENSION FL/2(Vz [m/s])  "Vz [m/s]"
  phi_dot [rad/s]1/1 -> SUSPENSION FL/4(phi_dot [rad/s])  "phi_dot [rad/s]"
  phi [rad]1/1 -> SUSPENSION FL/3(phi [rad])  "phi [rad]"
  theta [rad]1/1 -> SUSPENSION FL/5(theta [rad])  "theta [rad]"
  theta_dot [rad/s]1/1 -> SUSPENSION FL/6(theta_dot [rad/s])  "theta_dot [rad/s]"
  Bus Selector/1 -> SUSPENSION FR/8(yFR_road [m])  "<yFR_road [m]>"
  Bus Selector1/1 -> SUSPENSION FL/8(yFL_road [m])  "<yFL_road [m]>"

== system VDSE_2018b/14-DOF VEHICLE MODEL/SUSPENSION/Load Transfer ==
  note: OVERALL NORMAL FORCE CALCULATION
  note: DYNAMIC LOAD TRANSFER CALCULATION
  note: WEIGHT OF THE VEHICLE - CHECK
  ax [m/s^2] : Inport
  ay [m/s^2] : Inport  Port=2
  Tyre z Forces [N] : Inport  Port=3
  Add8 : Sum  Inputs=++++
  Bus Creator : BusCreator  Inputs=4
  Bus Selector : BusSelector  OutputSignals=fFLz [N],fFRz [N],fRLz [N],fRRz [N]
  Clock : Clock
  Constant : Constant  Value=(wF+wR)/2
  Constant1 : Constant  Value=lF+lR
  Coupling of load transfer and suspension reaction : Subsystem
  Delay : Delay  DelayLength=1
  Dynamic Lateral Load Transfer - Front : Subsystem
  Dynamic Lateral Load Transfer - Rear : Subsystem
  Dynamic Longitudinal Load Transfer : Subsystem
  Gain : Gain  Gain=1/9.81
  Scope : Scope
  Tire lift from the ground check : MATLAB Function  TreatAsAtomicUnit=on
  ax1 : InportShadow
  ay1 : InportShadow  Port=2
  Tyres z forces [N] : Outport
  wires:
  Bus Creator/1 -> Delay/1
  Tyre z Forces [N]/1 -> Bus Selector/1
  ay [m/s^2]/1 -> Dynamic Lateral Load Transfer - Rear/1(ay [m/s^2]), Dynamic Lateral Load Transfer - Front/1(ay [m/s^2])
  Add8/1 -> Gain/1
  Gain/1 -> Scope/1
  ax [m/s^2]/1 -> Dynamic Longitudinal Load Transfer/1(ax [m/s^2])
  Clock/1 -> Tire lift from the ground check/7(time)
  Tire lift from the ground check/1(FLz) -> [FL], Bus Creator/1  "FLz_Overall [N]"
  Tire lift from the ground check/2(FRz) -> [FR], Bus Creator/2  "FRz_Overall [N]"
  Tire lift from the ground check/3(RLz) -> [RL], Bus Creator/3  "RLz_Overall [N]"
  Tire lift from the ground check/4(RRz) -> [RR], Bus Creator/4  "RRz_Overall [N]"
  Constant/1 -> Tire lift from the ground check/8(trackwidth)
  Constant1/1 -> Tire lift from the ground check/9(wheelbase)
  ax1/1 -> Tire lift from the ground check/5(ax)
  ay1/1 -> Tire lift from the ground check/6(ay)
  [FL] -> Add8/1
  [FR] -> Add8/2
  [RL] -> Add8/3
  [RR] -> Add8/4
  Coupling of load transfer and suspension reaction/1(FLz_Overall [N]) -> Tire lift from the ground check/1(FLz_Overall)  "FLz_overall"
  Coupling of load transfer and suspension reaction/2(FRz_Overall [N]) -> Tire lift from the ground check/2(FRz_Overall)  "FRz_overall"
  Coupling of load transfer and suspension reaction/3(RLz_Overall [N]) -> Tire lift from the ground check/3(RLz_Overall)  "RLz_overall"
  Coupling of load transfer and suspension reaction/4(RRz_Overall [N]) -> Tire lift from the ground check/4(RRz_Overall)  "RRz_overall"
  Delay/1 -> Tyres z forces [N]/1
  Dynamic Longitudinal Load Transfer/1(Long. Dynamic Transfer [N]) -> Coupling of load transfer and suspension reaction/1(Longidutinal Load Transfer [N])
  Dynamic Lateral Load Transfer - Front/1(Lat. Dynamic Transfer [N]) -> Coupling of load transfer and suspension reaction/2(Lateral Load Transfer - Front [N])
  Dynamic Lateral Load Transfer - Rear/1(Lat. Dynamic Transfer [N]) -> Coupling of load transfer and suspension reaction/3(Lateral Load Transfer - Rear [N])
  Bus Selector/4 -> Coupling of load transfer and suspension reaction/7(<fRRz [N]>)  "<fRRz [N]>"
  Bus Selector/3 -> Coupling of load transfer and suspension reaction/6(<fRLz [N]>)  "<fRLz [N]>"
  Bus Selector/2 -> Coupling of load transfer and suspension reaction/5(<fFRz [N]>)  "<fFRz [N]>"
  Bus Selector/1 -> Coupling of load transfer and suspension reaction/4(<fFLz [N]>)  "<fFLz [N]>"

== system VDSE_2018b/14-DOF VEHICLE MODEL/SUSPENSION/REAR SUSPENSION ==
  z [m] : Inport
  Vz [m/s] : Inport  Port=2
  phi [rad] : Inport  Port=3
  phi_dot [rad/s] : Inport  Port=4
  theta [rad] : Inport  Port=5
  theta_dot [rad/s] : Inport  Port=6
  yrear_road [m] : Inport  Port=7
  Bus Selector : BusSelector  OutputSignals=yRR_road [m]
  Bus Selector1 : BusSelector  OutputSignals=yRL_road [m]
  SUSPENSION RL : Subsystem
  SUSPENSION RR : Subsystem
  Vz [m/s]1 : InportShadow  Port=2
  phi [rad]1 : InportShadow  Port=3
  phi_dot [rad/s]1 : InportShadow  Port=4
  theta [rad]1 : InportShadow  Port=5
  theta_dot [rad/s]1 : InportShadow  Port=6
  yrear_road [m]1 : InportShadow  Port=7
  z [m]1 : InportShadow
  fRRz [N] : Outport
  fRLz [N] : Outport  Port=2
  zRR [m] : Outport  Port=3
  zRR_dot [m/s] : Outport  Port=4
  zRL [m] : Outport  Port=5
  zRL_dot [m/s] : Outport  Port=6
  wires:
  yrear_road [m]1/1 -> Bus Selector1/1  "yrear_road [m]"
  yrear_road [m]/1 -> Bus Selector/1  "yrear_road [m]"
  [zRR] -> SUSPENSION RL/7(zRR [m])
  SUSPENSION RL/3(zRL [m]) -> [zRL], zRL [m]/1  "zRL [m]"
  SUSPENSION RL/2(zRL_dot [m/s]) -> [zRL_dot], zRL_dot [m/s]/1  "zRL_dot [m/s]"
  SUSPENSION RR/3(zRR_dot [m/s]) -> zRR_dot [m/s]/1, [zRR_dot]  "zRR_dot [m/s]"
  SUSPENSION RR/2(zRR [m]) -> [zRR], zRR [m]/1  "zRR [m]"
  SUSPENSION RR/1(fRRz [N]) -> fRRz [N]/1  "fRRz [N]"
  SUSPENSION RL/1(fRLz [N]) -> fRLz [N]/1  "fRLz [N]"
  [zRL] -> SUSPENSION RR/7(zRL [m])
  z [m]/1 -> SUSPENSION RR/1(z [m])  "z [m]"
  Vz [m/s]/1 -> SUSPENSION RR/2(Vz [m/s])  "Vz [m/s]"
  phi [rad]/1 -> SUSPENSION RR/3(phi [rad])  "phi [rad]"
  phi_dot [rad/s]/1 -> SUSPENSION RR/4(phi_dot [rad/s])  "phi_dot [rad/s]"
  theta [rad]/1 -> SUSPENSION RR/5(theta [rad])  "theta [rad]"
  theta_dot [rad/s]/1 -> SUSPENSION RR/6(theta_dot [rad/s])  "theta_dot [rad/s]"
  theta_dot [rad/s]1/1 -> SUSPENSION RL/6(theta_dot [rad/s])  "theta_dot [rad/s]"
  theta [rad]1/1 -> SUSPENSION RL/5(theta [rad])  "theta [rad]"
  phi_dot [rad/s]1/1 -> SUSPENSION RL/4(phi_dot [rad/s])  "phi_dot [rad/s]"
  Vz [m/s]1/1 -> SUSPENSION RL/2(Vz [m/s])  "Vz [m/s]"
  phi [rad]1/1 -> SUSPENSION RL/3(phi [rad])  "phi [rad]"
  z [m]1/1 -> SUSPENSION RL/1(z [m])  "z [m]"
  Bus Selector/1 -> SUSPENSION RR/8(yRR_road [m])  "<yRR_road [m]>"
  Bus Selector1/1 -> SUSPENSION RL/8(yRL_road [m])  "<yRL_road [m]>"

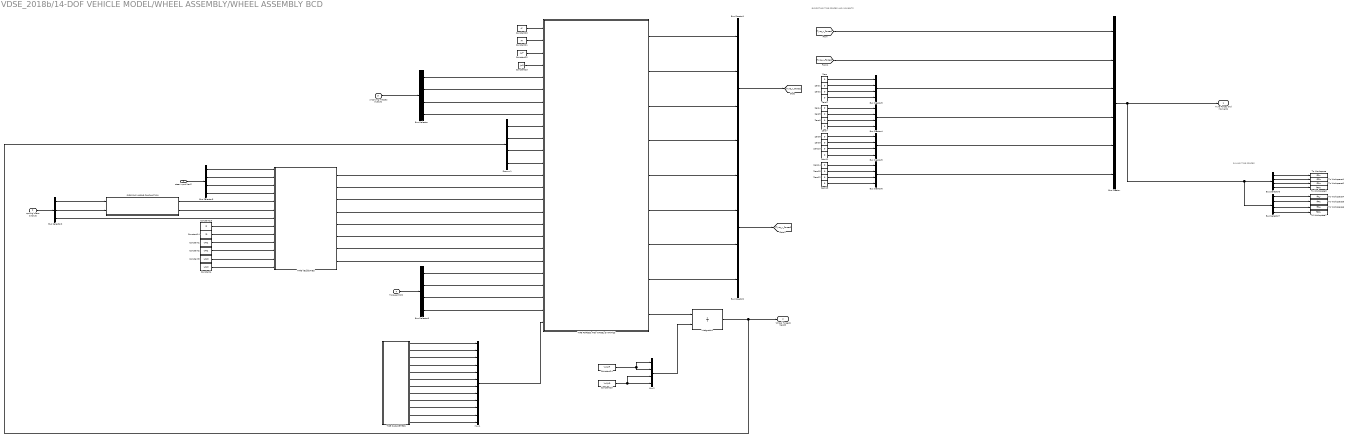
== system VDSE_2018b/14-DOF VEHICLE MODEL/WHEEL ASSEMBLY/WHEEL ASSEMBLY BCD ==
  note: EXPORTING TIRE FORCES AND MOMENTS
  note: SAVING TIRE FORCES
  steer input [rad] : Inport
  sprung mass outputs : Inport  Port=2
  unsprung masses outputs : Inport  Port=3
  Torques [Nm] : Inport  Port=4
  Bus Creator : BusCreator  Inputs=6
  Bus Creator{1..6} (6 alike) : BusCreator  Inputs=4
  Bus Selector : BusSelector  OutputSignals=Unsprung masses z Forces [N].FLz_Overall [N],Unsprung masses z Forces [N].FRz_Overall [N],Unsprung masses z Forces [N].RLz_Overall [N],Unsprung masses z Forces [N].RRz_Overall [N]
  Bus Selector2 : BusSelector  OutputSignals=Longitudinal Dynamics.Vx [m/s],Lateral Dynamics.Vy [m/s],Yaw dynamics.psi_dot [rad/s]
  Bus Selector3 : BusSelector  OutputSignals=Steering.deltaFL [rad],Steering.deltaFR [rad],Steering.deltaRL [rad],Steering.deltaRR [rad]
  Bus Selector5 : BusSelector  OutputSignals=TFL [Nm],TFR [Nm],TRL [Nm],TRR [Nm]
  Bus Selector6 : BusSelector  OutputSignals=Tyre x Forces [N].fFLx [N],Tyre x Forces [N].fFRx [N],Tyre x Forces [N].fRLx [N],Tyre x Forces [N].fRRx [N]
  Bus Selector7 : BusSelector  OutputSignals=Tyre y Forces [N].fFLy [N],Tyre y Forces [N].fFRy [N],Tyre y Forces [N].fRLy [N],Tyre y Forces [N].fRRy [N]
  Constant1 : Constant  Value=wF/2
  Constant13 : Constant  Value=lF
  Constant14 : Constant  Value=lR
  Constant2 : Constant  Value=wF/2
  Constant20 : Constant  Value=rF
  Constant21 : Constant  Value=rR
  Constant22 : Constant  Value=JwF
  Constant23 : Constant  Value=JwR
  Constant24 : Constant  Value=Vx0/rF
  Constant25 : Constant  Value=Vx0/rR
  Constant3 : Constant  Value=wR/2
  Constant4 : Constant  Value=wR/2
  Demux1 : Demux
  Integrator1 : Integrator  InitialConditionSource=external
  Mux1 : Mux  Inputs=12
  Mux2 : Mux
  SIDE SLIP ANGLE CALCULATION : Subsystem
  TIRE FORCES AND WHEEL DYNAMICS : MATLAB Function  TreatAsAtomicUnit=on
  TIRE PARAMETERS : Subsystem
  TIRE VELOCITIES : MATLAB Function  TreatAsAtomicUnit=on
  To Workspace : ToWorkspace  VariableName=fFLx  SaveFormat=Timeseries  SampleTime=-1
  To Workspace1 : ToWorkspace  VariableName=fFRx  SaveFormat=Timeseries  SampleTime=-1
  To Workspace2 : ToWorkspace  VariableName=fRLx  SaveFormat=Timeseries  SampleTime=-1
  To Workspace3 : ToWorkspace  VariableName=fRRx  SaveFormat=Timeseries  SampleTime=-1
  To Workspace4 : ToWorkspace  VariableName=fFLy  SaveFormat=Timeseries  SampleTime=-1
  To Workspace5 : ToWorkspace  VariableName=fFRy  SaveFormat=Timeseries  SampleTime=-1
  To Workspace6 : ToWorkspace  VariableName=fRLy  SaveFormat=Timeseries  SampleTime=-1
  To Workspace7 : ToWorkspace  VariableName=fRRy  SaveFormat=Timeseries  SampleTime=-1
  Zero{,1..15} (16 alike) : Constant  Value=0  OutDataTypeStr=Inherit: Inherit via back propagation
  Tyre Forces and Moments : Outport
  Wheel Speeds [rad/s] : Outport  Port=2
  wires:
  Bus Selector7/4 -> To Workspace7/1  "<fRRy [N]>"
  Bus Selector7/3 -> To Workspace6/1  "<fRLy [N]>"
  Bus Selector7/2 -> To Workspace5/1  "<fFRy [N]>"
  Bus Selector7/1 -> To Workspace4/1  "<fFLy [N]>"
  Bus Selector6/4 -> To Workspace3/1  "<fRRx [N]>"
  Bus Selector6/3 -> To Workspace2/1  "<fRLx [N]>"
  Bus Selector6/2 -> To Workspace1/1  "<fFRx [N]>"
  Bus Selector6/1 -> To Workspace/1  "<fFLx [N]>"
  Torques [Nm]/1 -> Bus Selector5/1
  Bus Creator/1 -> Tyre Forces and Moments/1, Bus Selector6/1, Bus Selector7/1
  steer input [rad]/1 -> Bus Selector3/1
  Bus Selector3/3 -> TIRE VELOCITIES/3(deltaRL)  "<deltaRL [rad]>"
  Bus Selector3/1 -> TIRE VELOCITIES/1(deltaFL)  "<deltaFL [rad]>"
  Bus Selector3/4 -> TIRE VELOCITIES/4(deltaRR)  "<deltaRR [rad]>"
  Bus Selector3/2 -> TIRE VELOCITIES/2(deltaFR)  "<deltaFR [rad]>"
  sprung mass outputs/1 -> Bus Selector2/1
  Bus Selector2/3 -> TIRE VELOCITIES/7(psidot)  "<psi_dot [rad/s]>"
  Bus Selector2/2 -> SIDE SLIP ANGLE CALCULATION/2(Vy [m/s])  "<Vy [m/s]>"
  Bus Selector2/1 -> SIDE SLIP ANGLE CALCULATION/1(Vx [m/s])  "<Vx [m/s]>"
  unsprung masses outputs/1 -> Bus Selector/1
  Bus Selector/2 -> TIRE FORCES AND WHEEL DYNAMICS/6(fFRz)  "<FRz_Overall [N]>"
  Bus Selector/3 -> TIRE FORCES AND WHEEL DYNAMICS/7(fRLz)  "<RLz_Overall [N]>"
  Bus Selector/4 -> TIRE FORCES AND WHEEL DYNAMICS/8(fRRz)  "<RRz_Overall [N]>"
  Bus Selector/1 -> TIRE FORCES AND WHEEL DYNAMICS/5(fFLz)  "<FLz_Overall [N]>"
  SIDE SLIP ANGLE CALCULATION/1(V [m/s]) -> TIRE VELOCITIES/5(V)  "V"
  SIDE SLIP ANGLE CALCULATION/2(beta [rad]) -> TIRE VELOCITIES/6(beta)  "beta"
  TIRE VELOCITIES/6(VRLy) -> TIRE FORCES AND WHEEL DYNAMICS/18(VRLy)  "VRLy"
  TIRE VELOCITIES/3(VFRx) -> TIRE FORCES AND WHEEL DYNAMICS/15(VFRx)  "VFRx"
  Constant3/1 -> TIRE VELOCITIES/12(wRL)
  TIRE VELOCITIES/5(VRLx) -> TIRE FORCES AND WHEEL DYNAMICS/17(VRLx)  "VRLx"
  Constant2/1 -> TIRE VELOCITIES/11(wFR)
  Constant14/1 -> TIRE VELOCITIES/9(lR)
  Constant1/1 -> TIRE VELOCITIES/10(wFL)
  Constant13/1 -> TIRE VELOCITIES/8(lF)
  Constant4/1 -> TIRE VELOCITIES/13(wRR)
  TIRE VELOCITIES/4(VFRy) -> TIRE FORCES AND WHEEL DYNAMICS/16(VFRy)  "VFRy"
  TIRE VELOCITIES/1(VFLx) -> TIRE FORCES AND WHEEL DYNAMICS/13(VFLx)  "VFLx"
  TIRE VELOCITIES/2(VFLy) -> TIRE FORCES AND WHEEL DYNAMICS/14(VFLy)  "VFLy"
  TIRE PARAMETERS/7(Byf) -> Mux1/7
  TIRE PARAMETERS/6(Dxr) -> Mux1/6
  TIRE PARAMETERS/12(Dyr) -> Mux1/12
  TIRE PARAMETERS/2(Cxf) -> Mux1/2
  Mux1/1 -> TIRE FORCES AND WHEEL DYNAMICS/25(TireParams)
  TIRE PARAMETERS/8(Cyf) -> Mux1/8
  TIRE PARAMETERS/9(Dyf) -> Mux1/9
  TIRE PARAMETERS/5(Cxr) -> Mux1/5
  TIRE PARAMETERS/3(Dxf) -> Mux1/3
  TIRE PARAMETERS/11(Cyr) -> Mux1/11
  TIRE PARAMETERS/10(Byr) -> Mux1/10
  TIRE PARAMETERS/4(Bxr) -> Mux1/4
  TIRE PARAMETERS/1(Bxf) -> Mux1/1
  Constant20/1 -> TIRE FORCES AND WHEEL DYNAMICS/1(rF)
  Constant22/1 -> TIRE FORCES AND WHEEL DYNAMICS/3(JwF)
  Constant23/1 -> TIRE FORCES AND WHEEL DYNAMICS/4(JwR)
  Constant21/1 -> TIRE FORCES AND WHEEL DYNAMICS/2(rR)
  Constant24/1 -> Mux2/2, Mux2/1
  Mux2/1 -> Integrator1/2
  Constant25/1 -> Mux2/3, Mux2/4
  TIRE FORCES AND WHEEL DYNAMICS/9(omega_dot) -> Integrator1/1  "omegas_dot [rad/s^2]"
  Demux1/1 -> TIRE FORCES AND WHEEL DYNAMICS/9(omegaFL)
  Demux1/2 -> TIRE FORCES AND WHEEL DYNAMICS/10(omegaFR)
  Demux1/3 -> TIRE FORCES AND WHEEL DYNAMICS/11(omegaRL)
  Demux1/4 -> TIRE FORCES AND WHEEL DYNAMICS/12(omegaRR)
  Integrator1/1 -> Demux1/1, Wheel Speeds [rad/s]/1  "omega [rad/s]"
  TIRE VELOCITIES/7(VRRx) -> TIRE FORCES AND WHEEL DYNAMICS/19(VRRx)  "VRRx"
  TIRE VELOCITIES/8(VRRy) -> TIRE FORCES AND WHEEL DYNAMICS/20(VRRy)  "VRRy"
  TIRE FORCES AND WHEEL DYNAMICS/6(fFRy) -> Bus Creator2/2  "fFRy [N]"
  TIRE FORCES AND WHEEL DYNAMICS/3(fRLx) -> Bus Creator1/3  "fRLx [N]"
  TIRE FORCES AND WHEEL DYNAMICS/4(fRRx) -> Bus Creator1/4  "fRRx [N]"
  Bus Creator1/1 -> [Tyre_x_Forces]  "Tyre x Forces [N]"
  TIRE FORCES AND WHEEL DYNAMICS/5(fFLy) -> Bus Creator2/1  "fFLy [N]"
  TIRE FORCES AND WHEEL DYNAMICS/7(fRLy) -> Bus Creator2/3  "fRLy [N]"
  TIRE FORCES AND WHEEL DYNAMICS/8(fRRy) -> Bus Creator2/4  "fRRy [N]"
  Bus Creator2/1 -> [Tyre_y_Forces]  "Tyre y Forces [N]"
  Zero6/1 -> Bus Creator4/3  "mRLx [Nm]"
  Zero3/1 -> Bus Creator3/4  "fRRz [N]"
  Zero5/1 -> Bus Creator4/2  "mFRx [Nm]"
  Zero7/1 -> Bus Creator4/4  "mRRx [Nm]"
  Zero1/1 -> Bus Creator3/2  "fFRz [N]"
  Zero4/1 -> Bus Creator4/1  "mFLx [Nm]"
  Zero2/1 -> Bus Creator3/3  "fRLz [N]"
  Zero/1 -> Bus Creator3/1  "fFLz [N]"
  Zero13/1 -> Bus Creator6/4  "mRRz [Nm]"
  Zero12/1 -> Bus Creator6/3  "mRLz [Nm]"
  Zero15/1 -> Bus Creator6/2  "mFRz [Nm]"
  Zero14/1 -> Bus Creator6/1  "mFLz [Nm]"
  TIRE FORCES AND WHEEL DYNAMICS/1(fFLx) -> Bus Creator1/1  "fFLx [N]"
  TIRE FORCES AND WHEEL DYNAMICS/2(fFRx) -> Bus Creator1/2  "fFRx [N]"
  [Tyre_x_Forces] -> Bus Creator/1  "Tyre x Forces [N]"
  [Tyre_y_Forces] -> Bus Creator/2  "Tyre y Forces [N]"
  Bus Creator3/1 -> Bus Creator/3  "Tyre z Forces [N]"
  Bus Creator4/1 -> Bus Creator/4  "Tyre Mx Moments [Nm]"
  Bus Creator5/1 -> Bus Creator/5  "Tyre My Moments [Nm]"
  Bus Creator6/1 -> Bus Creator/6  "Tyre Mz Moments [Nm]"
  Zero8/1 -> Bus Creator5/1  "mFLy [Nm]"
  Zero9/1 -> Bus Creator5/2  "mFRy [Nm]"
  Zero10/1 -> Bus Creator5/3  "mRLy [Nm]"
  Zero11/1 -> Bus Creator5/4  "mRRy [Nm]"
  Bus Selector5/1 -> TIRE FORCES AND WHEEL DYNAMICS/21(TFL)  "<TFL [Nm]>"
  Bus Selector5/2 -> TIRE FORCES AND WHEEL DYNAMICS/22(TFR)  "<TFR [Nm]>"
  Bus Selector5/3 -> TIRE FORCES AND WHEEL DYNAMICS/23(TRL)  "<TRL [Nm]>"
  Bus Selector5/4 -> TIRE FORCES AND WHEEL DYNAMICS/24(TRR)  "<TRR [Nm]>"
